simulink model "TrafficLight"  (R2021a)
settings: Solver=FixedStepAuto  StartTime=0.0  StopTime=10.0  RelTol=1e-3
settings Model: Creator=user  LastModifiedBy=user
settings OptimizationCC: DefaultParameterBehavior=Inlined  EnhancedBackFolding=on  PassReuseOutputArgsAs=Individual arguments  ZeroExternalMemoryAtStartup=off  ZeroInternalMemoryAtStartup=off  OptimizeBlockOrder=speed  DifferentSizesBufferReuse=on  OptimizationCustomize=off  EfficientTunableParamExpr=on
settings DebuggingCC: ParameterTunabilityLossMsg=error
settings SFSimCC: MATLABDynamicMemAlloc=off
settings RTWCC: SystemTargetFile=ert.tlc  GenCodeOnly=on  TemplateMakefile=ert_default_tmf  GenerateReport=on  IncludeHyperlinkInReport=on  LaunchReport=on  GenerateTraceInfo=on
settings CodeAppCC: ForceParamTrailComments=on  IgnoreCustomStorageClasses=off  OperatorAnnotations=on  SimulinkDataObjDesc=on  SFDataObjDesc=on  InsertBlockDesc=on
settings ERTTargetCC: TargetLangStandard=C99 (ISO)  GenerateSampleERTMain=on  InlinedParameterPlacement=NonHierarchical  ERTCustomFileTemplate=example_file_process.tlc

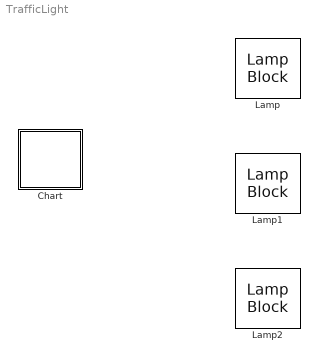
== system TrafficLight ==
  Chart : Stateflow chart  TreatAsAtomicUnit=on
  Lamp : LampBlock
  Lamp1 : LampBlock
  Lamp2 : LampBlock

== stateflow chart TrafficLight/Chart ==
  state Red
    entry: redLight=1;
    during: redTime=redTime+1;
    exit: redTime=0;
  state Yellow
    entry: yellowLight=1;
    during: yellowTime=yellowTime+1;
    exit: yellowTime=0;
  state Green
    entry: greenLight=1;
    during: greenTime=greenTime+1;
    exit: greenTime=0;
  (default) -> Red : {redTime=0;
      | greenTime=0;
      | yellowTime=0;}
  Yellow -> Red : [yellowTime>=50]{yellowLight=0;}
  Red -> Green : [redTime>=20]{redLight=0;}
  Green -> Yellow : [greenTime>=30
      | ]{greenLight=0;}
  data: redTime local; greenTime local; yellowTime local; redLight local; greenLight local; yellowLight local
